simulink model "PLL"  (R2022a)
settings: Solver=FixedStepAuto  StartTime=0.0  StopTime=3  FixedStep=Ts  RelTol=1e-3
values from neighbouring files (symbols this model uses):
  Cf = 0.001    [PLL_para.m]
  dt_jump = 2    [PLL_para.m]
  dt_sag = 0.01    [PLL_para.m]
  ki_pll1 = 0    [PLL_para.m]
  ki_pll2 = 0    [PLL_para.m]
  kp_pll1 = w_pll1    (= 62.8318530718)    [PLL_para.m]
  kp_pll2 = w_pll2    (= 62.8318530718)    [PLL_para.m]
  Lc = 1e-9    (= 1e-09)    [PLL_para.m]
  Lf = 0.2    [PLL_para.m]
  Lg0 = Xg    [PLL_para.m]
  Lg1 = X1    [PLL_para.m]
  Lg2 = X2    [PLL_para.m]
  phase_jump = -1.2    [PLL_para.m]
  position = position    [PLL_para.m]
  Rg0 = 0.1e-3    (= 0.0001)    [PLL_para.m]
  Rg1 = 0.1e-3    (= 0.0001)    [PLL_para.m]
  Rg2 = 0.1e-3    (= 0.0001)    [PLL_para.m]
  Sbase = 1    [PLL_para.m]
  t0 = 2    [PLL_para.m]
  t0_jump = 10    [PLL_para.m]
  t0_sag = 10    [PLL_para.m]
  tc1 = t_c    [PLL_para.m]
  tc2 = t_c    [PLL_para.m]
  Ts = 1/Fs    (= 1e-05)    [PLL_para.m]
  v_sag = 0.1    [PLL_para.m]
  Vbase = 1    [PLL_para.m]
  w_i_GFL1 = 4000 *2*pi    (= 25132.7412287)    [PLL_para.m]
  w_i_GFL2 = 4000 *2*pi    (= 25132.7412287)    [PLL_para.m]
  w_pll1 = 10 *2*pi    (= 62.8318530718)    [PLL_para.m]
  w_tau1 = 1e3 *2*pi    (= 6283.18530718)    [PLL_para.m]
  w_tau2 = 1e3 *2*pi    (= 6283.18530718)    [PLL_para.m]
  Wbase = 2*pi*50    (= 314.159265359)    [PLL_para.m]
  Zbase = Vbase/Ibase    (= 1)    [PLL_para.m]
undefined symbols (not defined in the file or in its folder): DiscIntNeverNeededParam, I1d, I1q, I2d, I2q, initial
libraries: spsVoltageMeasurementLib x60, spsCurrentMeasurementLib x54, spsThreePhaseSeriesRLCBranchLib x22, spsControlledVoltageSourceLib x18, spsSeriesRLCBranchLib x6, spsThreePhaseBreakerLib x4, spsMultimeterLib x2, spsThreePhaseFaultLib x2, spspowerguiLib x1
(part 1 of 4)
settings Model: Creator=admin_user  LastModifiedBy=yz7521
settings SolverCC: AlgebraicLoopSolver=TrustRegion
settings DataIOCC: ReturnWorkspaceOutputs=off
settings DebuggingCC: UnconnectedInputMsg=warning  UnconnectedOutputMsg=warning  UnconnectedLineMsg=warning  SFMachineParentedDataDiag=warning
settings RTWCC: DLArmComputeVersion=19.05

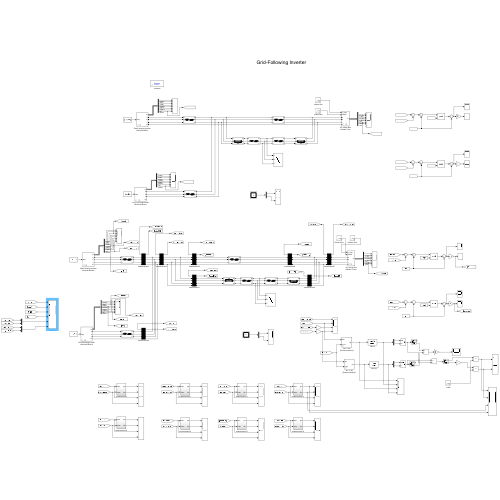
[thumbnail: Simulink's stored preview of the top-level diagram]
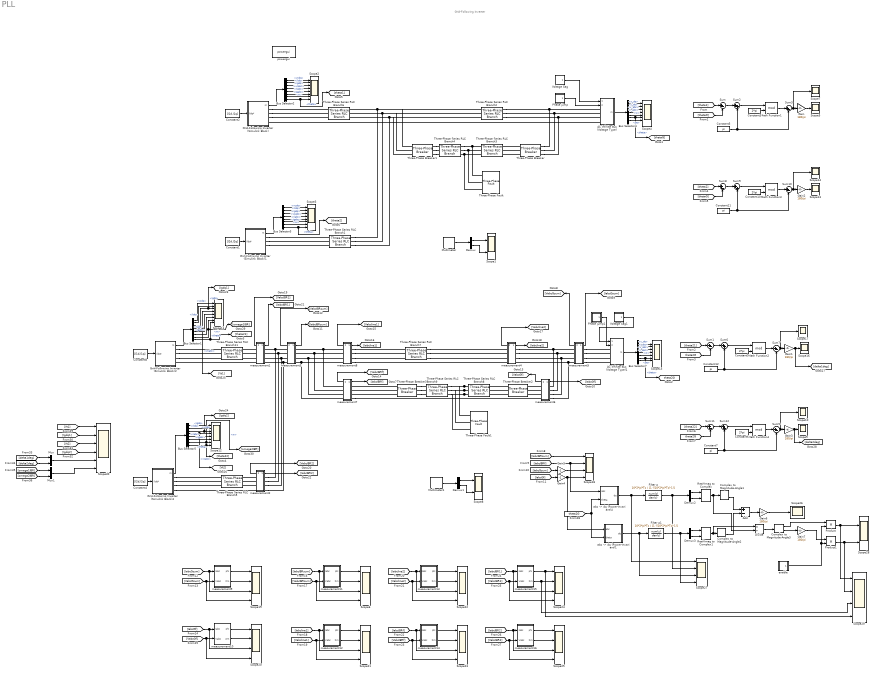
== system PLL ==
  note: Grid-Following Inverter
  AC Infinite Bus (Voltage Type) : Subsystem  AncestorBlock=|  mask{Ts=Ts, Sbase=Sbase, Vbase=Vbase, Wbase=Wbase, theta0=0, w=Wbase, R=1e-30}
      | SimplusGT/AC Infinite Bus
      | (Voltage Type)
      mask prompts: Ts "Ts (s), samping period"; Sbase "Sbase (VA), power base"; Vbase "Vbase (V), voltage base"; Wbase "Wbase (rad/s), frequency base"; theta0 "theta0 (rad), initial angle"; w "w (rad/s), frequency"; R "R (Ohm), resistance"
  AC Infinite Bus (Voltage Type)1 : Subsystem  AncestorBlock=|  mask{Ts=Ts, Sbase=Sbase, Vbase=Vbase, Wbase=Wbase, theta0=0, w=Wbase, R=1e-30}
      | SimplusGT/AC Infinite Bus
      | (Voltage Type)
      mask prompts: Ts "Ts (s), samping period"; Sbase "Sbase (VA), power base"; Vbase "Vbase (V), voltage base"; Wbase "Wbase (rad/s), frequency base"; theta0 "theta0 (rad), initial angle"; w "w (rad/s), frequency"; R "R (Ohm), resistance"
  Add : Sum  Inputs=+-
  Bus Selector{1..3,5} (4 alike) : BusSelector  OutputSignals=vcdq,ildq,igdq,vcabc,ilabc,igabc,w,theta
  Bus Selector4 : BusSelector  OutputSignals=v_dq,i_dq,v_abc,i_abc,w,theta,pq
  Bus Selector7 : BusSelector  OutputSignals=v_dq,i_dq,v_abc,i_abc,w,theta,pq
  Complex to Magnitude-Angle1 : ComplexToMagnitudeAngle
  Complex to Magnitude-Angle2 : ComplexToMagnitudeAngle
  Complex to Magnitude-Angle3 : ComplexToMagnitudeAngle
  Constant1 : Constant  Value=[I2d,I2q]
  Constant{3,6,9..10} (4 alike) : Constant  Value=2*pi
  Constant{5,7,11..12} (4 alike) : Constant  Value=pi
  Constant2 : Constant  Value=[I1d,I1q]
  Constant4 : Constant  Value=[I2d,I2q]
  Constant8 : Constant  Value=[I1d,I1q]
  Demux : Demux  Outputs=[3 3]
  Demux1 : Demux  Outputs=[3 3]
  Demux2 : Demux  Outputs=2
  Demux3 : Demux  Outputs=2
  Divide : Product  Inputs=*/
  Filter p : DiscreteTransferFcn  Numerator=10*2*pi*Ts  Denominator=[1 ((10*2*pi*Ts)-1)]  SampleTime=Ts
  Filter p1 : DiscreteTransferFcn  Numerator=10*2*pi*Ts  Denominator=[1 ((10*2*pi*Ts)-1)]  SampleTime=Ts
  Gain{,1..3,6..7} (6 alike) : Gain  Gain=180/pi
  Gain4 : Gain  Gain=-1
  Gain5 : Gain  Gain=-1
  Grid-Following Inverter (Simulink Block) : Subsystem  AncestorBlock=|  mask{Ts=Ts, Sbase=Sbase, Vbase=Vbase, Wbase=Wbase, w_i=w_i_GFL1, w_pll=w_pll1, w_tau=w_tau1, Lf=Lf, Cf=Cf, Lc=Lc}
      | SimplusGT/Grid-Following Inverter
      | (Simulink Block)
      mask prompts: Ts "Ts (s), sampling period"; Sbase "Sbase (VA), base power"; Vbase "Vbase (V), base voltage"; Wbase "Wbase (rad/s), base frequency"; w_i "w_i (rad/s), current-loop bandwidth"; w_pll "w_pll (rad/s), PLL bandwidth"; w_tau "w_tau (rad/s), PLL filter bandwidth"; Lf "Lf (pu), LCL filter"; Cf "Cf (pu), LCL filter"; Lc "Lc (pu), LCL filter"
  Grid-Following Inverter (Simulink Block)1 : Subsystem  AncestorBlock=|  mask{Ts=Ts, Sbase=Sbase, Vbase=Vbase, Wbase=Wbase, w_i=w_i_GFL2, w_pll=w_pll1, w_tau=w_tau1, Lf=Lf, Cf=Cf, Lc=Lc}
      | SimplusGT/Grid-Following Inverter
      | (Simulink Block)
      mask prompts: Ts "Ts (s), sampling period"; Sbase "Sbase (VA), base power"; Vbase "Vbase (V), base voltage"; Wbase "Wbase (rad/s), base frequency"; w_i "w_i (rad/s), current-loop bandwidth"; w_pll "w_pll (rad/s), PLL bandwidth"; w_tau "w_tau (rad/s), PLL filter bandwidth"; Lf "Lf (pu), LCL filter"; Cf "Cf (pu), LCL filter"; Lc "Lc (pu), LCL filter"
  Grid-Following Inverter (Simulink Block)2 : Subsystem  AncestorBlock=|  mask{Ts=Ts, Sbase=Sbase, Vbase=Vbase, Wbase=Wbase, w_i=w_i_GFL1, w_pll=w_pll1, w_tau=w_tau1, Lf=Lf, Cf=Cf, Lc=Lc}
      | SimplusGT/Grid-Following Inverter
      | (Simulink Block)
      mask prompts: Ts "Ts (s), sampling period"; Sbase "Sbase (VA), base power"; Vbase "Vbase (V), base voltage"; Wbase "Wbase (rad/s), base frequency"; w_i "w_i (rad/s), current-loop bandwidth"; w_pll "w_pll (rad/s), PLL bandwidth"; w_tau "w_tau (rad/s), PLL filter bandwidth"; Lf "Lf (pu), LCL filter"; Cf "Cf (pu), LCL filter"; Lc "Lc (pu), LCL filter"
  Grid-Following Inverter (Simulink Block)4 : Subsystem  AncestorBlock=|  mask{Ts=Ts, Sbase=Sbase, Vbase=Vbase, Wbase=Wbase, w_i=w_i_GFL2, w_pll=w_pll1, w_tau=w_tau1, Lf=Lf, Cf=Cf, Lc=Lc}
      | SimplusGT/Grid-Following Inverter
      | (Simulink Block)
      mask prompts: Ts "Ts (s), sampling period"; Sbase "Sbase (VA), base power"; Vbase "Vbase (V), base voltage"; Wbase "Wbase (rad/s), base frequency"; w_i "w_i (rad/s), current-loop bandwidth"; w_pll "w_pll (rad/s), PLL bandwidth"; w_tau "w_tau (rad/s), PLL filter bandwidth"; Lf "Lf (pu), LCL filter"; Cf "Cf (pu), LCL filter"; Lc "Lc (pu), LCL filter"
  Math Function{1..4} (4 alike) : Math  Operator=mod  SignedPower=on
  Multimeter : spsMultimeterLib/Multimeter  L=12  sel=[1 2 3 4 5 6]  yselected={}  Gain=[1 1 1 1 1 1]  OutputType=Complex  PlotAtSimulationStop=off  PhasorSimulation=off
  Multimeter1 : spsMultimeterLib/Multimeter  L=12  sel=[7 8 9 10 11 12]  yselected={}  Gain=[1 1 1 1 1 1]  OutputType=Complex  PlotAtSimulationStop=off  PhasorSimulation=off
  Mux : Mux  Inputs=2
  Mux1 : Mux  Inputs=2
  Phase jump : Subsystem  AncestorBlock=SimplusGT/Single Pulse  mask{t0=t0_jump, dt=dt_jump, Am=phase_jump}
      mask prompts: t0 "t0 (s), starting time"; dt "dt (s), pulse width"; Am "Am, pulse amplitude"
  Phase jump1 : Subsystem  AncestorBlock=SimplusGT/Single Pulse  mask{t0=t0_jump, dt=dt_jump, Am=phase_jump}
      mask prompts: t0 "t0 (s), starting time"; dt "dt (s), pulse width"; Am "Am, pulse amplitude"
  Product : Product
  Product1 : Product
  Real-Imag to Complex : RealImagToComplex
  Real-Imag to Complex1 : RealImagToComplex
  Scope1 : Scope  NumInputPorts=2
  Scope{5,7,9..10,13..14,16..17,26} (9 alike) : Scope
  Scope{2..4,11..12,15} (6 alike) : Scope  NumInputPorts=8
  Scope{6,18..25,27,29} (11 alike) : Scope  NumInputPorts=4
  Scope28 : Scope  NumInputPorts=2
  Scope30 : Scope  NumInputPorts=6
  Scope8 : Scope  NumInputPorts=2
  Sum{,1,3,5,7..8,10..11} (8 alike) : Sum  Inputs=|+-
  Sum{2,6,9,12} (4 alike) : Sum  Inputs=|++
  Three-Phase Series RLC Branch1 : spsThreePhaseSeriesRLCBranchLib/Three-Phase Series RLC Branch  LConnTagsString=A|B|C  RConnTagsString=A|B|C  BranchType=RL  Resistance=Rg2*Zbase  Inductance=Lg2*Zbase/Wbase  Capacitance=1/Wbase  Measurements=None
  Three-Phase Series RLC Branch11 : spsThreePhaseSeriesRLCBranchLib/Three-Phase Series RLC Branch  LConnTagsString=A|B|C  RConnTagsString=A|B|C  BranchType=RL  Resistance=Rg1*Zbase  Inductance=Lg1*Zbase/Wbase  Capacitance=1/Wbase  Measurements=None
  Three-Phase Series RLC Branch2 : spsThreePhaseSeriesRLCBranchLib/Three-Phase Series RLC Branch  LConnTagsString=A|B|C  RConnTagsString=A|B|C  BranchType=RL  Resistance=Rg0*Zbase  Inductance=Lg0*Zbase/Wbase  Capacitance=1/Wbase  Measurements=None
  Three-Phase Series RLC Branch3 : spsThreePhaseSeriesRLCBranchLib/Three-Phase Series RLC Branch  LConnTagsString=A|B|C  RConnTagsString=A|B|C  BranchType=RL  Resistance=Rg0*Zbase  Inductance=Lg0*Zbase/Wbase*position  Capacitance=1/Wbase  Measurements=None
  Three-Phase Series RLC Branch4 : spsThreePhaseSeriesRLCBranchLib/Three-Phase Series RLC Branch  LConnTagsString=A|B|C  RConnTagsString=A|B|C  BranchType=RL  Resistance=Rg0*Zbase  Inductance=Lg0*Zbase/Wbase*(1-position)  Capacitance=1/Wbase  Measurements=None
  Three-Phase Series RLC Branch5 : spsThreePhaseSeriesRLCBranchLib/Three-Phase Series RLC Branch  LConnTagsString=A|B|C  RConnTagsString=A|B|C  BranchType=RL  Resistance=Rg2*Zbase  Inductance=Lg2*Zbase/Wbase  Capacitance=1/Wbase  Measurements=None
  Three-Phase Series RLC Branch6 : spsThreePhaseSeriesRLCBranchLib/Three-Phase Series RLC Branch  LConnTagsString=A|B|C  RConnTagsString=A|B|C  BranchType=RL  Resistance=Rg1*Zbase  Inductance=Lg1*Zbase/Wbase  Capacitance=1/Wbase  Measurements=None
  Three-Phase Series RLC Branch7 : spsThreePhaseSeriesRLCBranchLib/Three-Phase Series RLC Branch  LConnTagsString=A|B|C  RConnTagsString=A|B|C  BranchType=RL  Resistance=Rg0*Zbase  Inductance=Lg0*Zbase/Wbase  Capacitance=1/Wbase  Measurements=None
  Three-Phase Series RLC Branch8 : spsThreePhaseSeriesRLCBranchLib/Three-Phase Series RLC Branch  LConnTagsString=A|B|C  RConnTagsString=A|B|C  BranchType=RL  Resistance=Rg0*Zbase  Inductance=Lg0*Zbase/Wbase*position  Capacitance=1/Wbase  Measurements=None
  Three-Phase Series RLC Branch9 : spsThreePhaseSeriesRLCBranchLib/Three-Phase Series RLC Branch  LConnTagsString=A|B|C  RConnTagsString=A|B|C  BranchType=RL  Resistance=Rg0*Zbase  Inductance=Lg0*Zbase/Wbase*(1-position)  Capacitance=1/Wbase  Measurements=None
  Three-Phase Breaker : spsThreePhaseBreakerLib/Three-Phase Breaker  InitialState=closed  SwitchA=on  SwitchB=on  SwitchC=on  SwitchTimes=[t0+tc1]  External=off  BreakerResistance=0.01e-3  SnubberResistance=1e8  SnubberCapacitance=inf  Measurements=Breaker currents
  Three-Phase Breaker1 : spsThreePhaseBreakerLib/Three-Phase Breaker  InitialState=closed  SwitchA=on  SwitchB=on  SwitchC=on  SwitchTimes=[t0+tc1]  External=off  BreakerResistance=0.01e-3  SnubberResistance=1e8  SnubberCapacitance=inf  Measurements=Breaker currents
  Three-Phase Breaker2 : spsThreePhaseBreakerLib/Three-Phase Breaker  InitialState=closed  SwitchA=on  SwitchB=on  SwitchC=on  SwitchTimes=[t0+tc2]  External=off  BreakerResistance=0.01e-3  SnubberResistance=1e8  SnubberCapacitance=inf  Measurements=Breaker currents
  Three-Phase Breaker3 : spsThreePhaseBreakerLib/Three-Phase Breaker  InitialState=closed  SwitchA=on  SwitchB=on  SwitchC=on  SwitchTimes=t0+tc2  External=off  BreakerResistance=0.01e-3  SnubberResistance=1e10  SnubberCapacitance=inf  Measurements=Breaker currents
  Three-Phase Fault : spsThreePhaseFaultLib/Three-Phase Fault  InitialStates=0  FaultA=on  FaultB=on  FaultC=on  GroundFault=on  SwitchTimes=[t0]  External=off  SwitchStatus=NaN  FaultResistance=Rf  GroundResistance=0.01e-6  SnubberResistance=10e6  SnubberCapacitance=inf  Measurements=None
  Three-Phase Fault1 : spsThreePhaseFaultLib/Three-Phase Fault  InitialStates=0  FaultA=on  FaultB=on  FaultC=on  GroundFault=on  SwitchTimes=[t0]  External=off  SwitchStatus=NaN  FaultResistance=Rf  GroundResistance=0.01e-6  SnubberResistance=10e6  SnubberCapacitance=inf  Measurements=None
  Voltage Sag : Subsystem  AncestorBlock=SimplusGT/Single Pulse  mask{t0=t0_sag, dt=dt_sag, Am=v_sag}
      mask prompts: t0 "t0 (s), starting time"; dt "dt (s), pulse width"; Am "Am, pulse amplitude"
  Voltage Sag1 : Subsystem  AncestorBlock=SimplusGT/Single Pulse  mask{t0=t0_sag, dt=dt_sag, Am=v_sag}
      mask prompts: t0 "t0 (s), starting time"; dt "dt (s), pulse width"; Am "Am, pulse amplitude"
  "abc -> dq (Power-Invariant)1" : Subsystem  AncestorBlock=|
      | SimplusGT/abc -> dq
      | (Power-Invariant)
  "abc -> dq (Power-Invariant)4" : Subsystem  AncestorBlock=|
      | SimplusGT/abc -> dq
      | (Power-Invariant)
  enable : Subsystem  AncestorBlock=SimplusGT/Single Pulse  mask{t0=0, dt=tc2+t0, Am=1}
      mask prompts: t0 "t0 (s), starting time"; dt "dt (s), pulse width"; Am "Am, pulse amplitude"
  measurement1 : Subsystem
      settings: PortSchema="{\"entries\":[{\"content\":{\"sides\":[{\"content\":{\"connectorIds\":[\"Out2\",\"LConn1\",\"LConn2\",\"LConn3\",\"LConn4\"]},\"type\":\"ConnectorPlacement.EquallySpacedRectSide\",\"uuid\":\"b97639c7-89ad-4c11-8fcc-ddc4f61f4533\"},{\"content\":{\"connectorIds\":[\"Out1\",\"RConn1\",\"RConn2\",\"RConn3\",\"RConn4\"],\"side\":\"RIGHT\"},\"type\":\"ConnectorPlacement.EquallySpacedRectSide\",\"uuid\":\"3b8f0759-83d7-4d3a-a5c5-bdf29e7cbe5b\"},{\"content\":{\"connectorIds\":[],\"side\":\"TOP\"},\"type\":\"ConnectorPlacement.EquallySpacedRectSide\",\"uuid\":\"1e391932-f1e1-4127-bfe0-28b7de5de667\"},{\"content\":{\"connectorIds\":[],\"side\":\"BOTTOM\"},\"type\":\"ConnectorPlacement.EquallySpacedRectSide\",\"uuid\":\"f0c236e9-048a-4270-a45f-ff2fecf0ec8b\"}]},\"type\":\"ConnectorPlacement.EquallySpacedConnector\",\"uuid\":\"002609f8-6c16-431f-ae58-b6d94c927972\"}],\"packageUris\":[\"http://schema.mathworks.com/mf0/Connector/R2020b\"],\"version\":\"1.0\"}"
  measurement10 : Subsystem
  measurement11 : Subsystem
  measurement12 : Subsystem
  measurement13 : Subsystem
  measurement14 : Subsystem
  measurement15 : Subsystem
  measurement16 : Subsystem
  measurement2 : Subsystem
      settings: PortSchema="{\"entries\":[{\"content\":{\"sides\":[{\"content\":{\"connectorIds\":[\"Out2\",\"LConn1\",\"LConn2\",\"LConn3\",\"LConn4\"]},\"type\":\"ConnectorPlacement.EquallySpacedRectSide\",\"uuid\":\"b97639c7-89ad-4c11-8fcc-ddc4f61f4533\"},{\"content\":{\"connectorIds\":[\"Out1\",\"RConn1\",\"RConn2\",\"RConn3\",\"RConn4\"],\"side\":\"RIGHT\"},\"type\":\"ConnectorPlacement.EquallySpacedRectSide\",\"uuid\":\"3b8f0759-83d7-4d3a-a5c5-bdf29e7cbe5b\"},{\"content\":{\"connectorIds\":[],\"side\":\"TOP\"},\"type\":\"ConnectorPlacement.EquallySpacedRectSide\",\"uuid\":\"1e391932-f1e1-4127-bfe0-28b7de5de667\"},{\"content\":{\"connectorIds\":[],\"side\":\"BOTTOM\"},\"type\":\"ConnectorPlacement.EquallySpacedRectSide\",\"uuid\":\"f0c236e9-048a-4270-a45f-ff2fecf0ec8b\"}]},\"type\":\"ConnectorPlacement.EquallySpacedConnector\",\"uuid\":\"002609f8-6c16-431f-ae58-b6d94c927972\"}],\"packageUris\":[\"http://schema.mathworks.com/mf0/Connector/R2020b\"],\"version\":\"1.0\"}"
  measurement3 : Subsystem
      settings: PortSchema="{\"entries\":[{\"content\":{\"sides\":[{\"content\":{\"connectorIds\":[\"Out2\",\"LConn1\",\"LConn2\",\"LConn3\",\"LConn4\"]},\"type\":\"ConnectorPlacement.EquallySpacedRectSide\",\"uuid\":\"b97639c7-89ad-4c11-8fcc-ddc4f61f4533\"},{\"content\":{\"connectorIds\":[\"Out1\",\"RConn1\",\"RConn2\",\"RConn3\",\"RConn4\"],\"side\":\"RIGHT\"},\"type\":\"ConnectorPlacement.EquallySpacedRectSide\",\"uuid\":\"3b8f0759-83d7-4d3a-a5c5-bdf29e7cbe5b\"},{\"content\":{\"connectorIds\":[],\"side\":\"TOP\"},\"type\":\"ConnectorPlacement.EquallySpacedRectSide\",\"uuid\":\"1e391932-f1e1-4127-bfe0-28b7de5de667\"},{\"content\":{\"connectorIds\":[],\"side\":\"BOTTOM\"},\"type\":\"ConnectorPlacement.EquallySpacedRectSide\",\"uuid\":\"f0c236e9-048a-4270-a45f-ff2fecf0ec8b\"}]},\"type\":\"ConnectorPlacement.EquallySpacedConnector\",\"uuid\":\"002609f8-6c16-431f-ae58-b6d94c927972\"}],\"packageUris\":[\"http://schema.mathworks.com/mf0/Connector/R2020b\"],\"version\":\"1.0\"}"
  measurement4 : Subsystem
      settings: PortSchema="{\"entries\":[{\"content\":{\"sides\":[{\"content\":{\"connectorIds\":[\"Out2\",\"LConn1\",\"LConn2\",\"LConn3\",\"LConn4\"]},\"type\":\"ConnectorPlacement.EquallySpacedRectSide\",\"uuid\":\"b97639c7-89ad-4c11-8fcc-ddc4f61f4533\"},{\"content\":{\"connectorIds\":[\"Out1\",\"RConn1\",\"RConn2\",\"RConn3\",\"RConn4\"],\"side\":\"RIGHT\"},\"type\":\"ConnectorPlacement.EquallySpacedRectSide\",\"uuid\":\"3b8f0759-83d7-4d3a-a5c5-bdf29e7cbe5b\"},{\"content\":{\"connectorIds\":[],\"side\":\"TOP\"},\"type\":\"ConnectorPlacement.EquallySpacedRectSide\",\"uuid\":\"1e391932-f1e1-4127-bfe0-28b7de5de667\"},{\"content\":{\"connectorIds\":[],\"side\":\"BOTTOM\"},\"type\":\"ConnectorPlacement.EquallySpacedRectSide\",\"uuid\":\"f0c236e9-048a-4270-a45f-ff2fecf0ec8b\"}]},\"type\":\"ConnectorPlacement.EquallySpacedConnector\",\"uuid\":\"002609f8-6c16-431f-ae58-b6d94c927972\"}],\"packageUris\":[\"http://schema.mathworks.com/mf0/Connector/R2020b\"],\"version\":\"1.0\"}"
  measurement5 : Subsystem
      settings: PortSchema="{\"entries\":[{\"content\":{\"sides\":[{\"content\":{\"connectorIds\":[\"Out2\",\"LConn1\",\"LConn2\",\"LConn3\",\"LConn4\"]},\"type\":\"ConnectorPlacement.EquallySpacedRectSide\",\"uuid\":\"b97639c7-89ad-4c11-8fcc-ddc4f61f4533\"},{\"content\":{\"connectorIds\":[\"Out1\",\"RConn1\",\"RConn2\",\"RConn3\",\"RConn4\"],\"side\":\"RIGHT\"},\"type\":\"ConnectorPlacement.EquallySpacedRectSide\",\"uuid\":\"3b8f0759-83d7-4d3a-a5c5-bdf29e7cbe5b\"},{\"content\":{\"connectorIds\":[],\"side\":\"TOP\"},\"type\":\"ConnectorPlacement.EquallySpacedRectSide\",\"uuid\":\"1e391932-f1e1-4127-bfe0-28b7de5de667\"},{\"content\":{\"connectorIds\":[],\"side\":\"BOTTOM\"},\"type\":\"ConnectorPlacement.EquallySpacedRectSide\",\"uuid\":\"f0c236e9-048a-4270-a45f-ff2fecf0ec8b\"}]},\"type\":\"ConnectorPlacement.EquallySpacedConnector\",\"uuid\":\"002609f8-6c16-431f-ae58-b6d94c927972\"}],\"packageUris\":[\"http://schema.mathworks.com/mf0/Connector/R2020b\"],\"version\":\"1.0\"}"
  measurement6 : Subsystem
      settings: PortSchema="{\"entries\":[{\"content\":{\"sides\":[{\"content\":{\"connectorIds\":[\"Out2\",\"LConn1\",\"LConn2\",\"LConn3\",\"LConn4\"]},\"type\":\"ConnectorPlacement.EquallySpacedRectSide\",\"uuid\":\"b97639c7-89ad-4c11-8fcc-ddc4f61f4533\"},{\"content\":{\"connectorIds\":[\"Out1\",\"RConn1\",\"RConn2\",\"RConn3\",\"RConn4\"],\"side\":\"RIGHT\"},\"type\":\"ConnectorPlacement.EquallySpacedRectSide\",\"uuid\":\"3b8f0759-83d7-4d3a-a5c5-bdf29e7cbe5b\"},{\"content\":{\"connectorIds\":[],\"side\":\"TOP\"},\"type\":\"ConnectorPlacement.EquallySpacedRectSide\",\"uuid\":\"1e391932-f1e1-4127-bfe0-28b7de5de667\"},{\"content\":{\"connectorIds\":[],\"side\":\"BOTTOM\"},\"type\":\"ConnectorPlacement.EquallySpacedRectSide\",\"uuid\":\"f0c236e9-048a-4270-a45f-ff2fecf0ec8b\"}]},\"type\":\"ConnectorPlacement.EquallySpacedConnector\",\"uuid\":\"002609f8-6c16-431f-ae58-b6d94c927972\"}],\"packageUris\":[\"http://schema.mathworks.com/mf0/Connector/R2020b\"],\"version\":\"1.0\"}"
  measurement7 : Subsystem
      settings: PortSchema="{\"entries\":[{\"content\":{\"sides\":[{\"content\":{\"connectorIds\":[\"Out2\",\"LConn1\",\"LConn2\",\"LConn3\",\"LConn4\"]},\"type\":\"ConnectorPlacement.EquallySpacedRectSide\",\"uuid\":\"b97639c7-89ad-4c11-8fcc-ddc4f61f4533\"},{\"content\":{\"connectorIds\":[\"Out1\",\"RConn1\",\"RConn2\",\"RConn3\",\"RConn4\"],\"side\":\"RIGHT\"},\"type\":\"ConnectorPlacement.EquallySpacedRectSide\",\"uuid\":\"3b8f0759-83d7-4d3a-a5c5-bdf29e7cbe5b\"},{\"content\":{\"connectorIds\":[],\"side\":\"TOP\"},\"type\":\"ConnectorPlacement.EquallySpacedRectSide\",\"uuid\":\"1e391932-f1e1-4127-bfe0-28b7de5de667\"},{\"content\":{\"connectorIds\":[],\"side\":\"BOTTOM\"},\"type\":\"ConnectorPlacement.EquallySpacedRectSide\",\"uuid\":\"f0c236e9-048a-4270-a45f-ff2fecf0ec8b\"}]},\"type\":\"ConnectorPlacement.EquallySpacedConnector\",\"uuid\":\"002609f8-6c16-431f-ae58-b6d94c927972\"}],\"packageUris\":[\"http://schema.mathworks.com/mf0/Connector/R2020b\"],\"version\":\"1.0\"}"
  measurement8 : Subsystem
      settings: PortSchema="{\"entries\":[{\"content\":{\"sides\":[{\"content\":{\"connectorIds\":[\"Out2\",\"LConn1\",\"LConn2\",\"LConn3\",\"LConn4\"]},\"type\":\"ConnectorPlacement.EquallySpacedRectSide\",\"uuid\":\"b97639c7-89ad-4c11-8fcc-ddc4f61f4533\"},{\"content\":{\"connectorIds\":[\"Out1\",\"RConn1\",\"RConn2\",\"RConn3\",\"RConn4\"],\"side\":\"RIGHT\"},\"type\":\"ConnectorPlacement.EquallySpacedRectSide\",\"uuid\":\"3b8f0759-83d7-4d3a-a5c5-bdf29e7cbe5b\"},{\"content\":{\"connectorIds\":[],\"side\":\"TOP\"},\"type\":\"ConnectorPlacement.EquallySpacedRectSide\",\"uuid\":\"1e391932-f1e1-4127-bfe0-28b7de5de667\"},{\"content\":{\"connectorIds\":[],\"side\":\"BOTTOM\"},\"type\":\"ConnectorPlacement.EquallySpacedRectSide\",\"uuid\":\"f0c236e9-048a-4270-a45f-ff2fecf0ec8b\"}]},\"type\":\"ConnectorPlacement.EquallySpacedConnector\",\"uuid\":\"002609f8-6c16-431f-ae58-b6d94c927972\"}],\"packageUris\":[\"http://schema.mathworks.com/mf0/Connector/R2020b\"],\"version\":\"1.0\"}"
  measurement9 : Subsystem
  powergui : spspowerguiLib/powergui  Priority=1  SimulationMode=Discrete  SampleTime=Ts  frequency=60  Iterations=50  frequencyindice=0  Pbase=100e6  ErrMax=1e-4  UnitsV=kV  UnitsW=MW  buscounter=0  FunctionMessages=off  echomessages=off  EnableUseOfTLC=off  CurrentSourceSwitches=off  DisableSnubberDevices=off  DisableRonSwitches=off  DisableVfSwitches=off  DisplayEquations=off  AutomaticDiscreteSolvers=off  SolverType=Tustin/Backward Euler (TBE)  Interpol=off  ExternalGateDelay=off  methode=off  Ts=100  x0status=blocks  SPID=on  SwTol=0  HookPort=off  NonlinearTolerance=1e-4  nMaxIteration=100  ContinueOnMaxIteration=off  RestoreLinks=warning  ResistiveCurrentMeasurement=off  Frange=[0:2:500]  Ylog=off  Xlog=on  ShowGrid=off  save=off  variable=ZData  structure=0  ZoomFFT=off  StartTime=0.0  cycles=1  DisplayStyle=1  fundamental=60  FreqAxis=off  MaxFrequency=1000  frequencyindicesteady=1  RmsSteady=1  display=off
  tag scope: theta2G=global
  wires:
  Bus Selector2/7 -> Scope2/7  "<w>"
  Bus Selector2/5 -> Scope2/5  "<ilabc>"
  Bus Selector2/6 -> Scope2/6  "<igabc>"
  Bus Selector2/3 -> Scope2/3  "<igdq>"
  Bus Selector2/8 -> [theta1], Scope2/8  "<theta>"
  Bus Selector2/4 -> Scope2/4  "<vcabc>"
  Bus Selector2/1 -> Scope2/1  "<vcdq>"
  Bus Selector2/2 -> Scope2/2  "<ildq>"
  Grid-Following Inverter (Simulink Block)/1(m) -> Bus Selector2/1
  Constant2/1 -> Grid-Following Inverter (Simulink Block)/1(ildq*)
  AC Infinite Bus (Voltage Type)/1(m) -> Bus Selector4/1
  Bus Selector4/1 -> Scope4/1  "<v_dq>"
  Bus Selector4/2 -> Scope4/2  "<i_dq>"
  Bus Selector4/4 -> Scope4/4  "<i_abc>"
  Bus Selector4/3 -> Scope4/3  "<v_abc>"
  Bus Selector4/5 -> Scope4/5  "<w>"
  Bus Selector4/6 -> [thetaG], Scope4/6  "<theta>"
  Bus Selector4/7 -> Scope4/7  "<pq>"
  Math Function1/1 -> Sum3/1
  Sum3/1 -> Scope7/1, Gain/1
  Sum2/1 -> Math Function1/1
  Constant3/1 -> Math Function1/2
  [thetaG] -> Sum/2
  [theta1] -> Sum/1
  Sum/1 -> Sum2/1
  Gain/1 -> Scope5/1
  Constant5/1 -> Sum2/2, Sum3/2
  [thetaG] -> Sum8/2
  Constant11/1 -> Sum9/2, Sum10/2
  Sum9/1 -> Math Function3/1
  Sum8/1 -> Sum9/1
  [theta2] -> Sum8/1
  Constant10/1 -> Math Function3/2
  Gain2/1 -> Scope13/1
  Bus Selector3/5 -> Scope3/5  "<ilabc>"
  Bus Selector3/3 -> Scope3/3  "<igdq>"
  Bus Selector3/4 -> Scope3/4  "<vcabc>"
  Math Function3/1 -> Sum10/1
  Sum10/1 -> Scope14/1, Gain2/1
  Bus Selector3/8 -> [theta2], Scope3/8  "<theta>"
  Bus Selector3/2 -> Scope3/2  "<ildq>"
  Grid-Following Inverter (Simulink Block)1/1(m) -> Bus Selector3/1
  Bus Selector3/6 -> Scope3/6  "<igabc>"
  Bus Selector3/7 -> Scope3/7  "<w>"
  Bus Selector3/1 -> Scope3/1  "<vcdq>"
  Constant1/1 -> Grid-Following Inverter (Simulink Block)1/1(ildq*)
  Phase jump/1(Out) -> AC Infinite Bus (Voltage Type)/2(Phase)
  Voltage Sag/1(Out) -> AC Infinite Bus (Voltage Type)/1(v_mag)
  Multimeter/1 -> Demux/1
  Demux/1 -> Scope1/1
  Demux/2 -> Scope1/2
  Multimeter1/1 -> Demux1/1
  Demux1/2 -> Scope8/2
  Constant7/1 -> Sum12/2, Sum5/2
  [theta21] -> Sum1/1
  Bus Selector1/7 -> [omega1IBR], Scope11/7  "<w>"
  Grid-Following Inverter (Simulink Block)2/1(m) -> Bus Selector1/1
  Bus Selector1/2 -> Scope11/2  "<ildq>"
  Sum12/1 -> Math Function4/1
  Bus Selector1/5 -> Scope11/5  "<ilabc>"
  Bus Selector5/6 -> Scope12/6  "<igabc>"
  Bus Selector5/2 -> Scope12/2  "<ildq>"
  Grid-Following Inverter (Simulink Block)4/1(m) -> Bus Selector5/1
  Constant4/1 -> Grid-Following Inverter (Simulink Block)4/1(ildq*)
  Bus Selector5/3 -> [Igdq2], Scope12/3  "<igdq>"
  [theta2G] -> Sum11/2
  Math Function4/1 -> Sum5/1
  Sum5/1 -> Scope10/1, Gain3/1
  Constant12/1 -> Sum6/2, Sum7/2
  Sum1/1 -> Sum6/1
  Bus Selector7/3 -> Scope15/3  "<v_abc>"
  Bus Selector5/5 -> Scope12/5  "<ilabc>"
  Gain3/1 -> [delta2deg], Scope9/1
  Constant6/1 -> Math Function4/2
  AC Infinite Bus (Voltage Type)1/1(m) -> Bus Selector7/1
  [theta22] -> Sum11/1
  Constant9/1 -> Math Function2/2
  [theta2G] -> Sum1/2
  Gain1/1 -> [delta1deg], Scope16/1
  Bus Selector1/6 -> Scope11/6  "<igabc>"
  Bus Selector7/4 -> Scope15/4  "<i_abc>"
  Bus Selector5/1 -> Scope12/1  "<vcdq>"
  Bus Selector7/5 -> Scope15/5  "<w>"
  Sum7/1 -> Scope17/1, Gain1/1
  Bus Selector5/7 -> [omega2IBR], Scope12/7  "<w>"
  Sum6/1 -> Math Function2/1
  Sum11/1 -> Sum12/1
  Voltage Sag1/1(Out) -> AC Infinite Bus (Voltage Type)1/1(v_mag)
  Math Function2/1 -> Sum7/1
  Bus Selector7/7 -> Scope15/7  "<pq>"
  Bus Selector7/6 -> [theta2G], Scope15/6  "<theta>"
  Bus Selector7/1 -> Scope15/1  "<v_dq>"
  Bus Selector1/4 -> [Vt1], Scope11/4  "<vcabc>"
  Bus Selector1/1 -> Scope11/1  "<vcdq>"
  Bus Selector1/3 -> [Igdq1], Scope11/3  "<igdq>"
  Constant8/1 -> Grid-Following Inverter (Simulink Block)2/1(ildq*)
  Phase jump1/1(Out) -> AC Infinite Bus (Voltage Type)1/2(Phase)
  Bus Selector7/2 -> Scope15/2  "<i_dq>"
  Bus Selector5/4 -> [Vt2], Scope12/4  "<vcabc>"
  Demux1/1 -> Scope8/1
  Bus Selector1/8 -> [theta21], Scope11/8  "<theta>"
  [IabcIBRsum] -> Scope18/1
  measurement6/1(Iabc) -> [IabcGf]
  [IabcGsum] -> Gain5/1
  [IabcGf] -> Gain4/1
  measurement3/1(Iabc) -> [IabcIBRsum]
  Bus Selector5/8 -> [theta22], Scope12/8  "<theta>"
  measurement7/1(Iabc) -> [IabcIBRf]
  measurement5/1(Iabc) -> [IabcGsum]
  measurement5/2(Vabc) -> [VabcGsum]
  measurement3/2(Vabc) -> [VabcIBRsum]
  measurement6/2(Vabc) -> [VabcGf]
  [VabcGsum] -> Scope19/4, measurement9/2(Vabc)
  measurement9/1(phi) -> Scope19/1
  measurement9/2(Zm) -> Scope19/2
  [IabcGsum] -> Scope19/3, measurement9/1(Iabc)
  [IabcGf] -> Scope20/3, measurement10/1(Iabc)
  measurement10/2(Zm) -> Scope20/2
  [VabcGf] -> Scope20/4, measurement10/2(Vabc)
  measurement10/1(phi) -> Scope20/1
  [IabcIBRsum] -> Scope6/3, measurement11/1(Iabc)
  measurement11/2(Zm) -> Scope6/2
  [VabcIBRsum] -> Scope6/4, measurement11/2(Vabc)
  measurement11/1(phi) -> Scope6/1
  [Iabcline1] -> Scope21/3, measurement12/1(Iabc)
  measurement12/2(Zm) -> Scope21/2
  [Vabcline1] -> Scope21/4, measurement12/2(Vabc)
  measurement12/1(phi) -> Scope21/1
  [Iabcline2] -> Scope22/3, measurement13/1(Iabc)
  measurement13/2(Zm) -> Scope22/2
  [Vabcline2] -> Scope22/4, measurement13/2(Vabc)
  measurement13/1(phi) -> Scope22/1
  [IabcIBRf] -> Scope23/3, measurement14/1(Iabc)
  measurement14/2(Zm) -> Scope23/2
  [VabcIBRf] -> Scope23/4, measurement14/2(Vabc)
  measurement14/1(phi) -> Scope23/1
  [IabcIBR1] -> Scope24/3, measurement15/1(Iabc)
  measurement15/2(Zm) -> Scope29/3, Scope24/2
  [VabcIBR1] -> Scope24/4, measurement15/2(Vabc)
  measurement15/1(phi) -> Scope29/4, Scope24/1
  [IabcIBR2] -> Scope25/3, measurement16/1(Iabc)
  measurement16/2(Zm) -> Scope25/2
  [VabcIBR2] -> Scope25/4, measurement16/2(Vabc)
  measurement16/1(phi) -> Scope25/1
  measurement7/2(Vabc) -> [VabcIBRf]
  measurement8/2(Vabc) -> [Vabcline1]
  measurement8/1(Iabc) -> [Iabcline1]
  measurement4/2(Vabc) -> [Vabcline2]
  measurement4/1(Iabc) -> [Iabcline2]
  measurement2/1(Iabc) -> [IabcIBR2]
  measurement2/2(Vabc) -> [VabcIBR2]
  measurement1/2(Vabc) -> [VabcIBR1]
  measurement1/1(Iabc) -> [IabcIBR1]
  Gain5/1 -> Scope18/3
  Gain6/1 -> Scope26/1
  Add/1 -> Gain6/1
  Demux3/2 -> Real-Imag to Complex1/2
  "abc -> dq (Power-Invariant)4"/1(dq) -> Scope27/1, Filter p/1
  [theta2G] -> "abc -> dq (Power-Invariant)4"/2(theta), "abc -> dq (Power-Invariant)1"/2(theta)
  Demux2/2 -> Real-Imag to Complex/2
  Demux3/1 -> Real-Imag to Complex1/1
  Gain4/1 -> "abc -> dq (Power-Invariant)1"/1(abc), Scope18/4
  Demux2/1 -> Real-Imag to Complex/1
  [IabcIBRf] -> "abc -> dq (Power-Invariant)4"/1(abc), Scope18/2
  Real-Imag to Complex/1 -> Divide/2, Complex to Magnitude-Angle1/1
  Real-Imag to Complex1/1 -> Divide/1, Complex to Magnitude-Angle2/1
  Complex to Magnitude-Angle1/2 -> Add/1
  Complex to Magnitude-Angle2/2 -> Add/2
  Filter p/1 -> Scope27/2, Demux2/1
  "abc -> dq (Power-Invariant)1"/1(dq) -> Scope27/3, Filter p1/1
  Filter p1/1 -> Scope27/4, Demux3/1
  Divide/1 -> Complex to Magnitude-Angle3/1
  Complex to Magnitude-Angle3/2 -> Gain7/1
  enable/1(Out) -> Product1/2, Product/2
  Complex to Magnitude-Angle3/1 -> Product/1
  Gain7/1 -> Product1/1
  Product/1 -> Scope29/1, Scope28/1
  Product1/1 -> Scope29/2, Scope28/2
  [Vt1] -> Scope30/1
  [Igdq1] -> Scope30/2
  [Vt2] -> Scope30/3
  [Igdq2] -> Scope30/4
  Mux/1 -> Scope30/5
  [delta1deg] -> Mux/1
  [delta2deg] -> Mux/2
  Mux1/1 -> Scope30/6
  [omega1IBR] -> Mux1/1
  [omega2IBR] -> Mux1/2
  connections:
  Grid-Following Inverter (Simulink Block)/RConn1 -- Three-Phase Series RLC Branch6/RConn1
  Grid-Following Inverter (Simulink Block)/RConn2 -- Three-Phase Series RLC Branch6/RConn2
  Grid-Following Inverter (Simulink Block)/RConn3 -- Three-Phase Series RLC Branch6/RConn3
  AC Infinite Bus (Voltage Type)/LConn4 -- Grid-Following Inverter (Simulink Block)/RConn4
  Three-Phase Series RLC Branch1/LConn1 -- Three-Phase Breaker1/LConn1 -- Three-Phase Series RLC Branch2/RConn1 -- Three-Phase Series RLC Branch6/LConn1
  Three-Phase Series RLC Branch1/LConn2 -- Three-Phase Breaker1/LConn2 -- Three-Phase Series RLC Branch2/RConn2 -- Three-Phase Series RLC Branch6/LConn2
  Three-Phase Series RLC Branch1/LConn3 -- Three-Phase Breaker1/LConn3 -- Three-Phase Series RLC Branch2/RConn3 -- Three-Phase Series RLC Branch6/LConn3
  Grid-Following Inverter (Simulink Block)1/RConn1 -- Three-Phase Series RLC Branch1/RConn1
  Grid-Following Inverter (Simulink Block)1/RConn3 -- Three-Phase Series RLC Branch1/RConn3
  Grid-Following Inverter (Simulink Block)1/RConn2 -- Three-Phase Series RLC Branch1/RConn2
  Three-Phase Series RLC Branch2/LConn1 -- Three-Phase Breaker/RConn1 -- AC Infinite Bus (Voltage Type)/LConn1
  Three-Phase Series RLC Branch2/LConn2 -- Three-Phase Breaker/RConn2 -- AC Infinite Bus (Voltage Type)/LConn2
  Three-Phase Series RLC Branch2/LConn3 -- Three-Phase Breaker/RConn3 -- AC Infinite Bus (Voltage Type)/LConn3
  Three-Phase Series RLC Branch4/LConn1 -- Three-Phase Fault/LConn1 -- Three-Phase Series RLC Branch3/RConn1
  Three-Phase Series RLC Branch4/LConn2 -- Three-Phase Fault/LConn2 -- Three-Phase Series RLC Branch3/RConn2
  Three-Phase Series RLC Branch4/LConn3 -- Three-Phase Fault/LConn3 -- Three-Phase Series RLC Branch3/RConn3
  Three-Phase Breaker/LConn1 -- Three-Phase Series RLC Branch3/LConn1
  Three-Phase Breaker/LConn2 -- Three-Phase Series RLC Branch3/LConn2
  Three-Phase Breaker/LConn3 -- Three-Phase Series RLC Branch3/LConn3
  Three-Phase Breaker1/RConn1 -- Three-Phase Series RLC Branch4/RConn1
  Three-Phase Breaker1/RConn2 -- Three-Phase Series RLC Branch4/RConn2
  Three-Phase Breaker1/RConn3 -- Three-Phase Series RLC Branch4/RConn3
  Three-Phase Series RLC Branch8/RConn1 -- Three-Phase Series RLC Branch9/LConn1 -- Three-Phase Fault1/LConn1
  Three-Phase Series RLC Branch8/RConn2 -- Three-Phase Series RLC Branch9/LConn2 -- Three-Phase Fault1/LConn2
  Three-Phase Series RLC Branch8/RConn3 -- Three-Phase Series RLC Branch9/LConn3 -- Three-Phase Fault1/LConn3
  Three-Phase Breaker3/LConn1 -- Three-Phase Series RLC Branch9/RConn3
  Three-Phase Breaker3/LConn3 -- Three-Phase Series RLC Branch9/RConn1
  Three-Phase Breaker3/LConn2 -- Three-Phase Series RLC Branch9/RConn2
  Grid-Following Inverter (Simulink Block)2/RConn1 -- Three-Phase Series RLC Branch11/RConn1
  Three-Phase Breaker2/LConn1 -- Three-Phase Series RLC Branch8/LConn1
  Grid-Following Inverter (Simulink Block)2/RConn3 -- Three-Phase Series RLC Branch11/RConn3
  Grid-Following Inverter (Simulink Block)4/RConn1 -- Three-Phase Series RLC Branch5/RConn1
  Three-Phase Breaker2/LConn3 -- Three-Phase Series RLC Branch8/LConn3
  Grid-Following Inverter (Simulink Block)4/RConn2 -- Three-Phase Series RLC Branch5/RConn2
  Grid-Following Inverter (Simulink Block)2/RConn2 -- Three-Phase Series RLC Branch11/RConn2
  Three-Phase Breaker2/LConn2 -- Three-Phase Series RLC Branch8/LConn2
  Grid-Following Inverter (Simulink Block)4/RConn3 -- Three-Phase Series RLC Branch5/RConn3
  measurement1/LConn1 -- Three-Phase Series RLC Branch11/LConn1
  measurement1/LConn2 -- Three-Phase Series RLC Branch11/LConn2
  measurement1/LConn3 -- Three-Phase Series RLC Branch11/LConn3
  measurement1/LConn4 -- Grid-Following Inverter (Simulink Block)2/RConn4
  measurement2/LConn1 -- Three-Phase Series RLC Branch5/LConn1
  measurement2/LConn2 -- Three-Phase Series RLC Branch5/LConn2
  measurement2/LConn3 -- Three-Phase Series RLC Branch5/LConn3
  measurement3/LConn1 -- measurement2/RConn1 -- measurement1/RConn1
  measurement3/LConn2 -- measurement2/RConn2 -- measurement1/RConn2
  measurement3/LConn3 -- measurement2/RConn3 -- measurement1/RConn3
  measurement3/LConn4 -- measurement1/RConn4 -- measurement2/RConn4
  measurement5/RConn4 -- AC Infinite Bus (Voltage Type)1/LConn4
  measurement5/LConn4 -- measurement6/RConn4 -- measurement4/RConn4
  Three-Phase Series RLC Branch7/LConn1 -- measurement4/LConn1
  Three-Phase Series RLC Branch7/LConn2 -- measurement4/LConn2
  Three-Phase Series RLC Branch7/LConn3 -- measurement4/LConn3
  measurement4/RConn1 -- measurement5/LConn1 -- measurement6/RConn1
  measurement4/RConn2 -- measurement5/LConn2 -- measurement6/RConn2
  measurement4/RConn3 -- measurement6/RConn3 -- measurement5/LConn3
  measurement5/RConn1 -- AC Infinite Bus (Voltage Type)1/LConn1
  measurement5/RConn2 -- AC Infinite Bus (Voltage Type)1/LConn2
  measurement5/RConn3 -- AC Infinite Bus (Voltage Type)1/LConn3
  measurement6/LConn1 -- Three-Phase Breaker2/RConn1
  measurement6/LConn2 -- Three-Phase Breaker2/RConn2
  measurement6/LConn3 -- Three-Phase Breaker2/RConn3
  Three-Phase Breaker3/RConn3 -- measurement7/RConn1
  Three-Phase Breaker3/RConn2 -- measurement7/RConn2
  Three-Phase Breaker3/RConn1 -- measurement7/RConn3
  measurement8/RConn1 -- Three-Phase Series RLC Branch7/RConn1
  measurement8/RConn2 -- Three-Phase Series RLC Branch7/RConn2
  measurement8/RConn3 -- Three-Phase Series RLC Branch7/RConn3
  measurement8/LConn1 -- measurement7/LConn1 -- measurement3/RConn1
  measurement8/LConn2 -- measurement7/LConn2 -- measurement3/RConn2
  measurement8/LConn3 -- measurement7/LConn3 -- measurement3/RConn3
  measurement8/LConn4 -- measurement7/LConn4 -- measurement3/RConn4
  measurement8/RConn4 -- measurement4/LConn4
  measurement7/RConn4 -- measurement6/LConn4
  Grid-Following Inverter (Simulink Block)4/RConn4 -- measurement2/LConn4

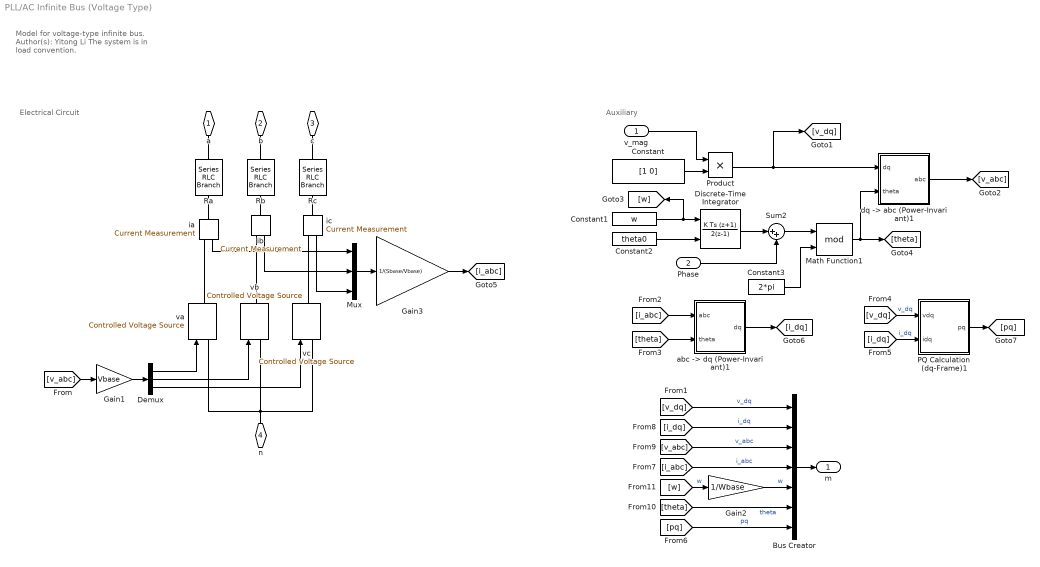
== system PLL/AC Infinite Bus (Voltage Type) ==
  note: Auxiliary
  note: Electrical Circuit
  note: Model for voltage-type infinite bus.
      |
      | Author(s): Yitong Li
      |
      | The system is in load convention.
  v_mag : Inport
  Phase : Inport  Port=2
  Bus Creator : BusCreator  Inputs=7
  Constant : Constant  Value=[1 0]
  Constant1 : Constant  Value=w
  Constant2 : Constant  Value=theta0
  Constant3 : Constant  Value=2*pi
  Demux : Demux  Outputs=3
  Discrete-Time Integrator : DiscreteIntegrator  IntegratorMethod=Integration: Trapezoidal  InitialConditionSource=external  SampleTime=-1  ICPrevOutput=DiscIntNeverNeededParam  ICPrevScaledInput=DiscIntNeverNeededParam
  Gain1 : Gain  Gain=Vbase
  Gain2 : Gain  Gain=1/Wbase
  Gain3 : Gain  Gain=1/(Sbase/Vbase)
  Math Function1 : Math  Operator=mod  SignedPower=on
  Mux : Mux  Inputs=3
  PQ Calculation (dq-Frame)1 : Subsystem  AncestorBlock=|
      | SimplusGT/PQ Calculation
      | (dq-Frame)
  Product : Product
  Ra : spsSeriesRLCBranchLib/Series RLC Branch  LConnTagsString=__new0  RConnTagsString=__new0  BranchType=R  Resistance=R  Inductance=1e-3  SetiL0=off  InitialCurrent=0  Capacitance=1e-6  Setx0=off  InitialVoltage=0  Measurements=None
  Rb : spsSeriesRLCBranchLib/Series RLC Branch  LConnTagsString=__new0  RConnTagsString=__new0  BranchType=R  Resistance=R  Inductance=1e-3  SetiL0=off  InitialCurrent=0  Capacitance=1e-6  Setx0=off  InitialVoltage=0  Measurements=None
  Rc : spsSeriesRLCBranchLib/Series RLC Branch  LConnTagsString=__new0  RConnTagsString=__new0  BranchType=R  Resistance=R  Inductance=1e-3  SetiL0=off  InitialCurrent=0  Capacitance=1e-6  Setx0=off  InitialVoltage=0  Measurements=None
  Sum2 : Sum  Inputs=|++
  "abc -> dq (Power-Invariant)1" : Subsystem  AncestorBlock=|
      | SimplusGT/abc -> dq
      | (Power-Invariant)
  "dq -> abc (Power-Invariant)1" : Subsystem  AncestorBlock=|
      | SimplusGT/dq -> abc
      | (Power-Invariant)
  ia : spsCurrentMeasurementLib/Current Measurement  PhasorSimulation=off  OutputType=Complex  PSBequivalent=0
  ib : spsCurrentMeasurementLib/Current Measurement  PhasorSimulation=off  OutputType=Complex  PSBequivalent=0
  ic : spsCurrentMeasurementLib/Current Measurement  PhasorSimulation=off  OutputType=Complex  PSBequivalent=0
  va : spsControlledVoltageSourceLib/Controlled Voltage Source  Initialize=on  Source_Type=AC  Amplitude=0  Phase=0  Frequency=0  Measurements=None
  vb : spsControlledVoltageSourceLib/Controlled Voltage Source  Initialize=on  Source_Type=AC  Amplitude=0  Phase=0  Frequency=0  Measurements=None
  vc : spsControlledVoltageSourceLib/Controlled Voltage Source  Initialize=on  Source_Type=AC  Amplitude=0  Phase=0  Frequency=0  Measurements=None
  a : PMIOPort  Side=Left
  b : PMIOPort  Port=2  Side=Left
  c : PMIOPort  Port=3  Side=Left
  n : PMIOPort  Port=4  Side=Left
  m : Outport
  wires:
  [pq] -> Bus Creator/7  "pq"
  PQ Calculation (dq-Frame)1/1(pq) -> [pq]
  [i_dq] -> PQ Calculation (dq-Frame)1/2(idq)  "i_dq"
  [v_dq] -> PQ Calculation (dq-Frame)1/1(vdq)  "v_dq"
  Gain3/1 -> [i_abc]
  Mux/1 -> Gain3/1
  Gain1/1 -> Demux/1
  "abc -> dq (Power-Invariant)1"/1(dq) -> [i_dq]
  [theta] -> "abc -> dq (Power-Invariant)1"/2(theta)
  [i_abc] -> "abc -> dq (Power-Invariant)1"/1(abc)
  ic/1 -> Mux/3
  ib/1 -> Mux/2
  ia/1 -> Mux/1
  [theta] -> Bus Creator/6  "theta"
  Bus Creator/1 -> m/1
  [i_dq] -> Bus Creator/2  "i_dq"
  Gain2/1 -> Bus Creator/5  "w"
  [v_abc] -> Bus Creator/3  "v_abc"
  [w] -> Gain2/1  "w"
  [i_abc] -> Bus Creator/4  "i_abc"
  [v_dq] -> Bus Creator/1  "v_dq"
  Constant3/1 -> Math Function1/2
  "dq -> abc (Power-Invariant)1"/1(abc) -> [v_abc]
  Constant1/1 -> [w], Discrete-Time Integrator/1
  Constant2/1 -> Discrete-Time Integrator/2
  Math Function1/1 -> [theta], "dq -> abc (Power-Invariant)1"/2(theta)
  Demux/3 -> vc/1
  Demux/2 -> vb/1
  Demux/1 -> va/1
  [v_abc] -> Gain1/1
  Constant/1 -> Product/2
  v_mag/1 -> Product/1
  Product/1 -> [v_dq], "dq -> abc (Power-Invariant)1"/1(dq)
  Discrete-Time Integrator/1 -> Sum2/1
  Sum2/1 -> Math Function1/1
  Phase/1 -> Sum2/2
  connections:
  Rc/LConn1 -- c/RConn1
  Rc/RConn1 -- ic/LConn1
  Rb/LConn1 -- b/RConn1
  ib/LConn1 -- Rb/RConn1
  Ra/LConn1 -- a/RConn1
  Ra/RConn1 -- ia/LConn1
  ic/RConn1 -- vc/RConn1
  ib/RConn1 -- vb/RConn1
  ia/RConn1 -- va/RConn1
  vb/LConn1 -- va/LConn1 -- n/RConn1 -- vc/LConn1

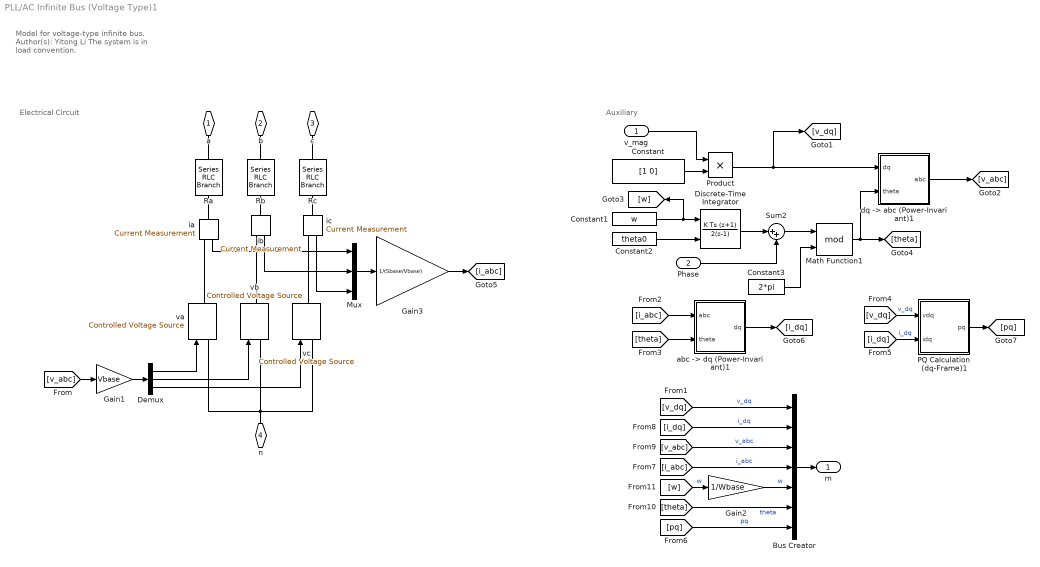
== system PLL/AC Infinite Bus (Voltage Type)1 ==
  note: Auxiliary
  note: Electrical Circuit
  note: Model for voltage-type infinite bus.
      |
      | Author(s): Yitong Li
      |
      | The system is in load convention.
  v_mag : Inport
  Phase : Inport  Port=2
  Bus Creator : BusCreator  Inputs=7
  Constant : Constant  Value=[1 0]
  Constant1 : Constant  Value=w
  Constant2 : Constant  Value=theta0
  Constant3 : Constant  Value=2*pi
  Demux : Demux  Outputs=3
  Discrete-Time Integrator : DiscreteIntegrator  IntegratorMethod=Integration: Trapezoidal  InitialConditionSource=external  SampleTime=-1  ICPrevOutput=DiscIntNeverNeededParam  ICPrevScaledInput=DiscIntNeverNeededParam
  Gain1 : Gain  Gain=Vbase
  Gain2 : Gain  Gain=1/Wbase
  Gain3 : Gain  Gain=1/(Sbase/Vbase)
  Math Function1 : Math  Operator=mod  SignedPower=on
  Mux : Mux  Inputs=3
  PQ Calculation (dq-Frame)1 : Subsystem  AncestorBlock=|
      | SimplusGT/PQ Calculation
      | (dq-Frame)
  Product : Product
  Ra : spsSeriesRLCBranchLib/Series RLC Branch  LConnTagsString=__new0  RConnTagsString=__new0  BranchType=R  Resistance=R  Inductance=1e-3  SetiL0=off  InitialCurrent=0  Capacitance=1e-6  Setx0=off  InitialVoltage=0  Measurements=None
  Rb : spsSeriesRLCBranchLib/Series RLC Branch  LConnTagsString=__new0  RConnTagsString=__new0  BranchType=R  Resistance=R  Inductance=1e-3  SetiL0=off  InitialCurrent=0  Capacitance=1e-6  Setx0=off  InitialVoltage=0  Measurements=None
  Rc : spsSeriesRLCBranchLib/Series RLC Branch  LConnTagsString=__new0  RConnTagsString=__new0  BranchType=R  Resistance=R  Inductance=1e-3  SetiL0=off  InitialCurrent=0  Capacitance=1e-6  Setx0=off  InitialVoltage=0  Measurements=None
  Sum2 : Sum  Inputs=|++
  "abc -> dq (Power-Invariant)1" : Subsystem  AncestorBlock=|
      | SimplusGT/abc -> dq
      | (Power-Invariant)
  "dq -> abc (Power-Invariant)1" : Subsystem  AncestorBlock=|
      | SimplusGT/dq -> abc
      | (Power-Invariant)
  ia : spsCurrentMeasurementLib/Current Measurement  PhasorSimulation=off  OutputType=Complex  PSBequivalent=0
  ib : spsCurrentMeasurementLib/Current Measurement  PhasorSimulation=off  OutputType=Complex  PSBequivalent=0
  ic : spsCurrentMeasurementLib/Current Measurement  PhasorSimulation=off  OutputType=Complex  PSBequivalent=0
  va : spsControlledVoltageSourceLib/Controlled Voltage Source  Initialize=on  Source_Type=AC  Amplitude=0  Phase=0  Frequency=0  Measurements=None
  vb : spsControlledVoltageSourceLib/Controlled Voltage Source  Initialize=on  Source_Type=AC  Amplitude=0  Phase=0  Frequency=0  Measurements=None
  vc : spsControlledVoltageSourceLib/Controlled Voltage Source  Initialize=on  Source_Type=AC  Amplitude=0  Phase=0  Frequency=0  Measurements=None
  a : PMIOPort  Side=Left
  b : PMIOPort  Port=2  Side=Left
  c : PMIOPort  Port=3  Side=Left
  n : PMIOPort  Port=4  Side=Left
  m : Outport
  wires:
  [pq] -> Bus Creator/7  "pq"
  PQ Calculation (dq-Frame)1/1(pq) -> [pq]
  [i_dq] -> PQ Calculation (dq-Frame)1/2(idq)  "i_dq"
  [v_dq] -> PQ Calculation (dq-Frame)1/1(vdq)  "v_dq"
  Gain3/1 -> [i_abc]
  Mux/1 -> Gain3/1
  Gain1/1 -> Demux/1
  "abc -> dq (Power-Invariant)1"/1(dq) -> [i_dq]
  [theta] -> "abc -> dq (Power-Invariant)1"/2(theta)
  [i_abc] -> "abc -> dq (Power-Invariant)1"/1(abc)
  ic/1 -> Mux/3
  ib/1 -> Mux/2
  ia/1 -> Mux/1
  [theta] -> Bus Creator/6  "theta"
  Bus Creator/1 -> m/1
  [i_dq] -> Bus Creator/2  "i_dq"
  Gain2/1 -> Bus Creator/5  "w"
  [v_abc] -> Bus Creator/3  "v_abc"
  [w] -> Gain2/1  "w"
  [i_abc] -> Bus Creator/4  "i_abc"
  [v_dq] -> Bus Creator/1  "v_dq"
  Constant3/1 -> Math Function1/2
  "dq -> abc (Power-Invariant)1"/1(abc) -> [v_abc]
  Constant1/1 -> [w], Discrete-Time Integrator/1
  Constant2/1 -> Discrete-Time Integrator/2
  Math Function1/1 -> [theta], "dq -> abc (Power-Invariant)1"/2(theta)
  Demux/3 -> vc/1
  Demux/2 -> vb/1
  Demux/1 -> va/1
  [v_abc] -> Gain1/1
  Constant/1 -> Product/2
  v_mag/1 -> Product/1
  Product/1 -> [v_dq], "dq -> abc (Power-Invariant)1"/1(dq)
  Discrete-Time Integrator/1 -> Sum2/1
  Sum2/1 -> Math Function1/1
  Phase/1 -> Sum2/2
  connections:
  Rc/LConn1 -- c/RConn1
  Rc/RConn1 -- ic/LConn1
  Rb/LConn1 -- b/RConn1
  ib/LConn1 -- Rb/RConn1
  Ra/LConn1 -- a/RConn1
  Ra/RConn1 -- ia/LConn1
  ic/RConn1 -- vc/RConn1
  ib/RConn1 -- vb/RConn1
  ia/RConn1 -- va/RConn1
  vb/LConn1 -- va/LConn1 -- n/RConn1 -- vc/LConn1

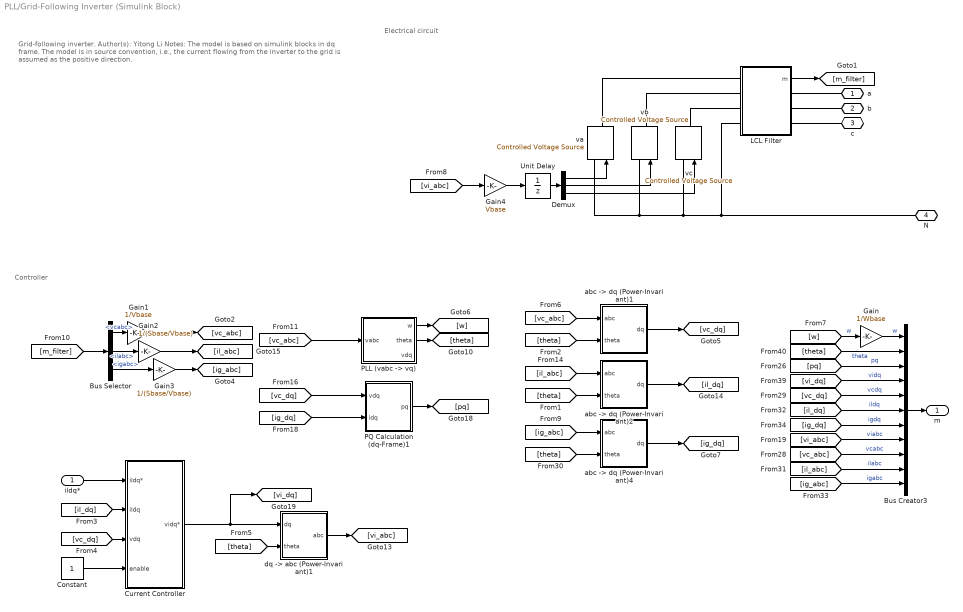
== system PLL/Grid-Following Inverter (Simulink Block) ==
  note: Grid-following inverter.
      |
      | Author(s): Yitong Li
      |
      | Notes:
      |
      | The model is based on simulink blocks in dq frame.
      |
      | The model is in source convention, i.e., the current flowing from the inverter to the grid is assumed as the positive direction.
  note: Electrical circuit
  note: Controller
  ildq* : Inport
  Bus Creator3 : BusCreator  Inputs=11
  Bus Selector : BusSelector  OutputSignals=vcabc,ilabc,igabc
  Constant : Constant
  Current Controller : Subsystem  mask{Ts=Ts, Wbase=Wbase, Lf=Lf/Wbase, Kg=0, Kp=w_i*Lf/Wbase, Ki=w_i*w_i/4*Lf/Wbase, vdmax=inf, vqmax=inf, Kcd=0}
      mask prompts: Ts "Sampling Time (s)"; Wbase "Base Angular Frequency (rad/s)"; Lf "Inductance"; Kg "Estimator Gain"; Kp "Proportional Gain"; Ki "Integral Gain"; vdmax "Voltage D Limit"; vqmax "Voltage Q Limit"; Kcd "Cross Decoupling Gain"
  Demux : Demux  Outputs=3
  Gain : Gain  Gain=1/Wbase
  Gain1 : Gain  Gain=1/Vbase
  Gain2 : Gain  Gain=1/(Sbase/Vbase)
  Gain3 : Gain  Gain=1/(Sbase/Vbase)
  Gain4 : Gain  Gain=Vbase
  LCL Filter : Subsystem  AncestorBlock=SimplexPS/LCL Filter  mask{Lf=Lf*(Vbase^2/Sbase)/Wbase, Rf=Lf*(Vbase^2/Sbase)/5, Lc=Lc*(Vbase^2/Sbase)/Wbase, Rc=Lc*(Vbase^2/Sbase)/5, Cf=Cf*(Sbase/Vbase^2)/Wbase, Rd=1e-5*(Vbase^2/Sbase)}
      mask prompts: Lf "Lf (H)"; Rf "Rf (Ohm)"; Lc "Lc (H)"; Rc "Rc (Ohm)"; Cf "Cf (F)"; Rd "Rd (Ohm)"
  "PLL (vabc -> vq)" : Subsystem  AncestorBlock=|  mask{Ts=Ts, Vbase=Vbase, Wbase=Wbase, kp=kp_pll1, ki=ki_pll1, w_tau=w_tau1, theta0=0}
      | SimplusGT/PLL
      | (vabc -> vq)
      mask prompts: Ts "Ts (s), sampling period"; Vbase "Vbase (V), base voltage"; Wbase "Wbase (rad/s), base angular frequency"; kp "PLL Proportional Gain"; ki "PLL Integral Gain"; w_tau "w_tau (rad/s), low-pass filter bandwidth"; theta0 "theta0 (rad), initial angle"
  PQ Calculation (dq-Frame)1 : Subsystem  AncestorBlock=|
      | SimplusGT/PQ Calculation
      | (dq-Frame)
  Unit Delay : UnitDelay  SampleTime=-1  HasFrameUpgradeWarning=on
  "abc -> dq (Power-Invariant)1" : Subsystem  AncestorBlock=|
      | SimplusGT/abc -> dq
      | (Power-Invariant)
  "abc -> dq (Power-Invariant)2" : Subsystem  AncestorBlock=|
      | SimplusGT/abc -> dq
      | (Power-Invariant)
  "abc -> dq (Power-Invariant)4" : Subsystem  AncestorBlock=|
      | SimplusGT/abc -> dq
      | (Power-Invariant)
  "dq -> abc (Power-Invariant)1" : Subsystem  AncestorBlock=|
      | SimplusGT/dq -> abc
      | (Power-Invariant)
  va : spsControlledVoltageSourceLib/Controlled Voltage Source  Initialize=on  Source_Type=AC  Amplitude=0  Phase=0  Frequency=0  Measurements=None
  vb : spsControlledVoltageSourceLib/Controlled Voltage Source  Initialize=on  Source_Type=AC  Amplitude=0  Phase=0  Frequency=0  Measurements=None
  vc : spsControlledVoltageSourceLib/Controlled Voltage Source  Initialize=on  Source_Type=AC  Amplitude=0  Phase=0  Frequency=0  Measurements=None
  a : PMIOPort  Side=Right
  b : PMIOPort  Port=2  Side=Right
  c : PMIOPort  Port=3  Side=Right
  N : PMIOPort  Port=4  Side=Right
  m : Outport
  wires:
  [vi_abc] -> Gain4/1
  Gain4/1 -> Unit Delay/1
  Gain3/1 -> [ig_abc]
  Gain2/1 -> [il_abc]
  Gain1/1 -> [vc_abc]
  [ig_abc] -> Bus Creator3/11  "igabc"
  [il_abc] -> Bus Creator3/10  "ilabc"
  [vc_abc] -> Bus Creator3/9  "vcabc"
  [vi_abc] -> Bus Creator3/8  "viabc"
  [ig_dq] -> Bus Creator3/7  "igdq"
  [il_dq] -> Bus Creator3/6  "ildq"
  [vc_dq] -> Bus Creator3/5  "vcdq"
  [vi_dq] -> Bus Creator3/4  "vidq"
  [pq] -> Bus Creator3/3  "pq"
  [theta] -> Bus Creator3/2  "theta"
  Gain/1 -> Bus Creator3/1  "w"
  [w] -> Gain/1  "w"
  Bus Selector/1 -> Gain1/1  "<vcabc>"
  Unit Delay/1 -> Demux/1
  [m_filter] -> Bus Selector/1
  "abc -> dq (Power-Invariant)2"/1(dq) -> [il_dq]
  "abc -> dq (Power-Invariant)4"/1(dq) -> [ig_dq]
  "abc -> dq (Power-Invariant)1"/1(dq) -> [vc_dq]
  [vc_abc] -> "PLL (vabc -> vq)"/1(vabc)
  [il_dq] -> Current Controller/2(iIdq)
  ildq*/1 -> Current Controller/1(iIdq*)
  [ig_dq] -> PQ Calculation (dq-Frame)1/2(idq)
  PQ Calculation (dq-Frame)1/1(pq) -> [pq]
  [vc_dq] -> PQ Calculation (dq-Frame)1/1(vdq)
  [theta] -> "dq -> abc (Power-Invariant)1"/2(theta)
  Current Controller/1(vidq*) -> [vi_dq], "dq -> abc (Power-Invariant)1"/1(dq)
  [vc_dq] -> Current Controller/3(vdq)
  Constant/1 -> Current Controller/4(enable)
  "PLL (vabc -> vq)"/1(w) -> [w]
  "PLL (vabc -> vq)"/2(theta) -> [theta]
  Bus Selector/2 -> Gain2/1  "<ilabc>"
  Bus Selector/3 -> Gain3/1  "<igabc>"
  [theta] -> "abc -> dq (Power-Invariant)4"/2(theta)
  [ig_abc] -> "abc -> dq (Power-Invariant)4"/1(abc)
  [il_abc] -> "abc -> dq (Power-Invariant)2"/1(abc)
  [vc_abc] -> "abc -> dq (Power-Invariant)1"/1(abc)
  [theta] -> "abc -> dq (Power-Invariant)2"/2(theta)
  [theta] -> "abc -> dq (Power-Invariant)1"/2(theta)
  Demux/3 -> vc/1
  Demux/2 -> vb/1
  Demux/1 -> va/1
  LCL Filter/1(m) -> [m_filter]
  Bus Creator3/1 -> m/1
  "dq -> abc (Power-Invariant)1"/1(abc) -> [vi_abc]
  connections:
  LCL Filter/LConn3 -- vc/RConn1
  va/LConn1 -- vb/LConn1 -- vc/LConn1 -- LCL Filter/LConn4 -- N/RConn1
  LCL Filter/RConn3 -- c/RConn1
  LCL Filter/RConn2 -- b/RConn1
  LCL Filter/RConn1 -- a/RConn1
  LCL Filter/LConn1 -- va/RConn1
  LCL Filter/LConn2 -- vb/RConn1
